simulink model "associative"  (R2024a)
settings: Solver=VariableStepAuto  StartTime=0.0  StopTime=10.0  RelTol=1e-3
settings Model: Creator=tusha  LastModifiedBy=tusha

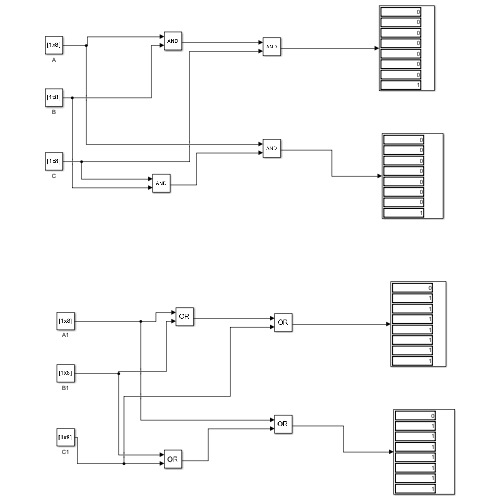
[thumbnail: Simulink's stored preview of the top-level diagram]
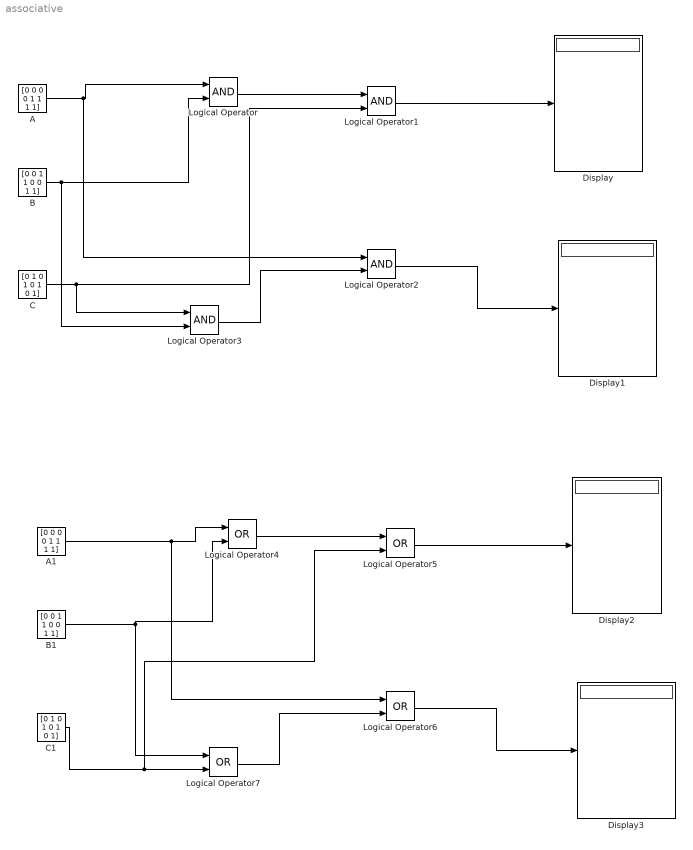
== system associative ==
  A : Constant  Value=[0 0 0 0 1 1 1 1]
  A1 : Constant  Value=[0 0 0 0 1 1 1 1]
  B : Constant  Value=[0 0 1 1 0 0 1 1]
  B1 : Constant  Value=[0 0 1 1 0 0 1 1]
  C : Constant  Value=[0 1 0 1 0 1 0 1]
  C1 : Constant  Value=[0 1 0 1 0 1 0 1]
  Display{,1..3} (4 alike) : Display
  Logical Operator{,1..3} (4 alike) : Logic  AllPortsSameDT=off  OutDataTypeStr=boolean
  Logical Operator{4..7} (4 alike) : Logic  Operator=OR  AllPortsSameDT=off  OutDataTypeStr=boolean
  wires:
  A/1 -> Logical Operator2/1, Logical Operator/1
  Logical Operator/1 -> Logical Operator1/1
  B/1 -> Logical Operator3/2, Logical Operator/2
  C/1 -> Logical Operator3/1, Logical Operator1/2
  Logical Operator1/1 -> Display/1
  Logical Operator3/1 -> Logical Operator2/2
  Logical Operator2/1 -> Display1/1
  Logical Operator7/1 -> Logical Operator6/2
  A1/1 -> Logical Operator4/1, Logical Operator6/1
  C1/1 -> Logical Operator5/2, Logical Operator7/2
  B1/1 -> Logical Operator7/1, Logical Operator4/2
  Logical Operator5/1 -> Display2/1
  Logical Operator6/1 -> Display3/1
  Logical Operator4/1 -> Logical Operator5/1
